simulink model "hard_threshold_adaptive"  (R2019b)
settings: Solver=VariableStepAuto  StartTime=0.0  StopTime=10  RelTol=1e-3
libraries: dspswit3 x1, dspstat3 x1, simulink x1
settings Model: Creator=sbuccelli  LastModifiedBy=sbuccelli

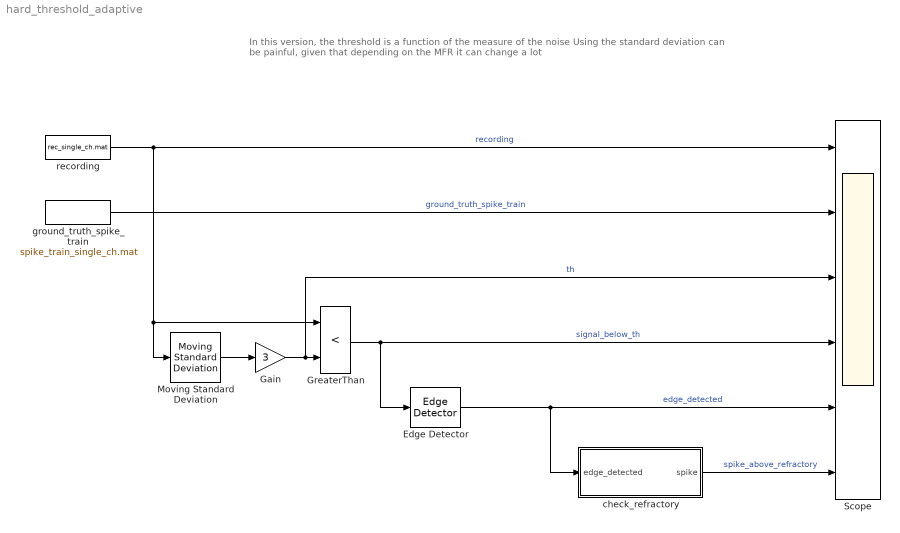
== system hard_threshold_adaptive ==
  note: In this version, the threshold is a function of the measure of the noise
      |
      | Using the standard deviation can be painful, given that depending on the MFR it can
      | change a lot
  Edge Detector : dspswit3/Edge Detector  InputProcessing=Columns as channels (frame based)
      settings: SourceProductName=DSP System Toolbox  SourceProductBaseCode=DS
  Gain : Gain  Gain=3
  GreaterThan : RelationalOperator  Operator=<  OutDataTypeStr=boolean  RndMeth=Simplest
  Moving Standard Deviation : dspstat3/Moving Standard Deviation  Method=Sliding window  ForgettingFactorPort=off  SpecifyWindowLength=on  WindowLength=3200  ForgettingFactor=0.9  SimulateUsing=Code generation
      settings: SourceProductName=DSP System Toolbox  SourceProductBaseCode=DS
  Scope : Scope  NumInputPorts=6
  check_refractory : Subsystem
  ground_truth_spike_train : FromFile  FileName=spike_train_single_ch.mat  SampleTime=1/32e3
  recording : FromFile  FileName=rec_single_ch.mat  SampleTime=1/32e3
  wires:
  recording/1 -> Scope/1, GreaterThan/1, Moving Standard Deviation/1  "recording"
  ground_truth_spike_train/1 -> Scope/2  "ground_truth_spike_train"
  Moving Standard Deviation/1 -> Gain/1
  Edge Detector/1 -> Scope/5, check_refractory/1(edge_detected)  "edge_detected"
  check_refractory/1(spike) -> Scope/6  "spike_above_refractory"
  GreaterThan/1 -> Scope/4, Edge Detector/1  "signal_below_th"
  Gain/1 -> Scope/3, GreaterThan/2  "th"

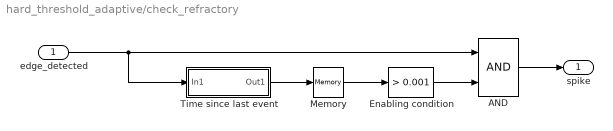
== system hard_threshold_adaptive/check_refractory ==
  edge_detected : Inport
  AND : Logic  IconShape=distinctive  AllPortsSameDT=off  OutDataTypeStr=boolean
  Enabling condition : simulink/Logic and Bit Operations/Compare To Constant  relop=>  const=0.001  OutDataTypeStr=boolean
  Memory : Memory  InheritSampleTime=on
  "Time since last event " : Subsystem
  spike : Outport
  wires:
  edge_detected/1 -> "Time since last event "/1(In1), AND/1
  Enabling condition/1 -> AND/2
  Memory/1 -> Enabling condition/1
  "Time since last event "/1(Out1) -> Memory/1
  AND/1 -> spike/1

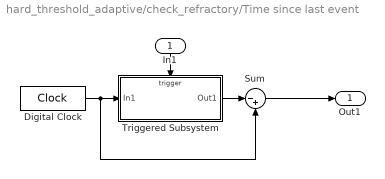
== system hard_threshold_adaptive/check_refractory/Time since last event  ==
  In1 : Inport
  Digital Clock : DigitalClock  SampleTime=1/32e3
  Sum : Sum  Inputs=|-+
  Triggered Subsystem : Subsystem  TreatAsAtomicUnit=on
  Out1 : Outport
  wires:
  Digital Clock/1 -> Sum/2, Triggered Subsystem/1(In1)
  Triggered Subsystem/1(Out1) -> Sum/1
  In1/1 -> Triggered Subsystem/Trigger
  Sum/1 -> Out1/1

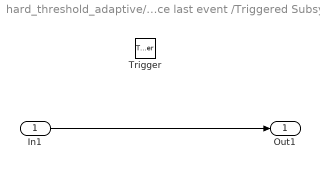
== system hard_threshold_adaptive/check_refractory/Time since last event /Triggered Subsystem ==
  In1 : Inport
  Trigger : TriggerPort  VariantControl=Variant
  Out1 : Outport
  wires:
  In1/1 -> Out1/1
